simulink model "prueba3"  (R2021a)
settings: Solver=VariableStepAuto  StartTime=0.0  StopTime=inf  RelTol=1e-3
libraries: slDxl_lib x11, simulink x1
settings Model: Creator=johnc  LastModifiedBy=johnc

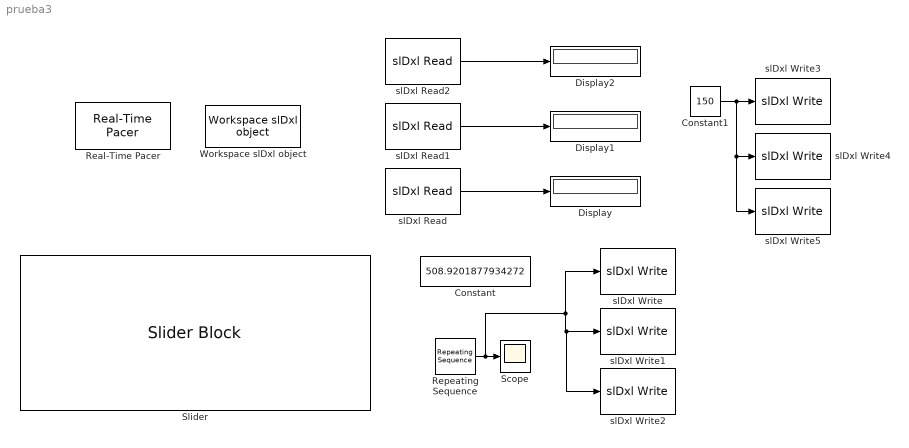
== system prueba3 ==
  Constant : Constant  Value=508.9201877934272
  Constant1 : Constant  Value=150
  Display : Display
  Display1 : Display
  Display2 : Display
  Real-Time Pacer : slDxl_lib/Real-Time Pacer  simTimePerRealTime=1
  Repeating Sequence : simulink/Sources/Repeating Sequence  rep_seq_t=[0 5]  rep_seq_y=[256 768]
  Scope : Scope
  Slider : SliderBlock  ScaleMax=1024
  Workspace slDxl object : slDxl_lib/Workspace slDxl object  slDxlVarName=Existing Object Handle #1  workspaceVarName=myDxl
  slDxl Read : slDxl_lib/slDxl Read  slDxlObject=Existing Object Handle #1  DXL_ID=3  DXL_ADDR=36  DXL_READ_SIZE=2  sampleT=Ts
  slDxl Read1 : slDxl_lib/slDxl Read  slDxlObject=Existing Object Handle #1  DXL_ID=2  DXL_ADDR=36  DXL_READ_SIZE=2  sampleT=Ts
  slDxl Read2 : slDxl_lib/slDxl Read  slDxlObject=Existing Object Handle #1  DXL_ID=1  DXL_ADDR=36  DXL_READ_SIZE=2  sampleT=Ts
  slDxl Write : slDxl_lib/slDxl Write  slDxlObject=Existing Object Handle #1  DXL_ID=1  DXL_ADDR=30  DXL_WRITE_SIZE=2  sampleT=Ts
  slDxl Write1 : slDxl_lib/slDxl Write  slDxlObject=Existing Object Handle #1  DXL_ID=2  DXL_ADDR=30  DXL_WRITE_SIZE=2  sampleT=Ts
  slDxl Write2 : slDxl_lib/slDxl Write  slDxlObject=Existing Object Handle #1  DXL_ID=3  DXL_ADDR=30  DXL_WRITE_SIZE=2  sampleT=Ts
  slDxl Write3 : slDxl_lib/slDxl Write  slDxlObject=Existing Object Handle #1  DXL_ID=1  DXL_ADDR=32  DXL_WRITE_SIZE=2  sampleT=Ts
  slDxl Write4 : slDxl_lib/slDxl Write  slDxlObject=Existing Object Handle #1  DXL_ID=2  DXL_ADDR=32  DXL_WRITE_SIZE=2  sampleT=Ts
  slDxl Write5 : slDxl_lib/slDxl Write  slDxlObject=Existing Object Handle #1  DXL_ID=3  DXL_ADDR=32  DXL_WRITE_SIZE=2  sampleT=Ts
  wires:
  slDxl Read/1 -> Display/1
  Constant1/1 -> slDxl Write5/1, slDxl Write4/1, slDxl Write3/1
  slDxl Read1/1 -> Display1/1
  slDxl Read2/1 -> Display2/1
  Repeating Sequence/1 -> slDxl Write2/1, slDxl Write1/1, slDxl Write/1, Scope/1
